simulink model "PID_Pointing"  (R2022b)
settings: Solver=VariableStepAuto  StartTime=0.0  StopTime=10.0  RelTol=1e-3
undefined symbols (not defined in the file): Kd, Ki, Kp
settings Model: Creator=Ze'ev Krischer  LastModifiedBy=Ze'ev Krischer

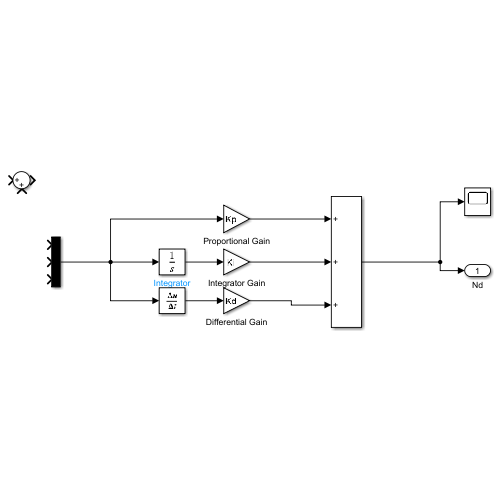
[thumbnail: Simulink's stored preview of the top-level diagram]
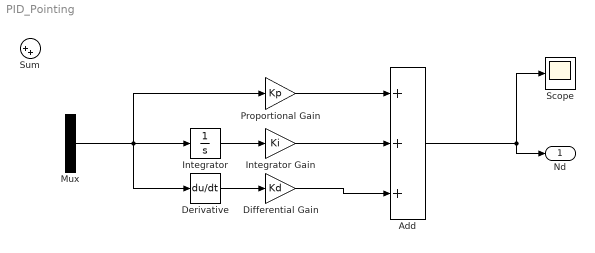
== system PID_Pointing ==
  Add : Sum  Inputs=+++
  Derivative : Derivative
  Differential Gain : Gain  Gain=Kd
  Integrator : Integrator
  Integrator Gain : Gain  Gain=Ki
  Mux : Mux  Inputs=3
  Proportional Gain : Gain  Gain=Kp
  Scope : Scope
  Sum : Sum  Inputs=|++
  Nd : Outport
  wires:
  Add/1 -> Nd/1, Scope/1
  Integrator/1 -> Integrator Gain/1
  Derivative/1 -> Differential Gain/1
  Proportional Gain/1 -> Add/1
  Integrator Gain/1 -> Add/2
  Differential Gain/1 -> Add/3
  Mux/1 -> Derivative/1, Integrator/1, Proportional Gain/1
